simulink model "Engine_TestBench"  (R2017a)
settings: Solver=VariableStepAuto  StartTime=0.0  StopTime=1700  FixedStep=0.01  RelTol=1e-3  EnableMultiTasking=on
PostLoadFcn:
  | , if any(exist('dsrtsu_mdlpostloadfcn', 'file') == [2, 3, 6]), try dsrtsu_mdlpostloadfcn('Execute', bdroot); catch fprintf('Error in PostLoadFcn (dsrtsu_mdlpostloadfcn) for model "%s":\n %s\n', bdroot, lasterr); end, end,
undefined symbols (not defined in the file): air, Engine, env, max_vehicle_rad_air_flow, NeutralGear, ParkGear
libraries: Pneumatic_lib x24, simulink x18, nesl_utility x18, EC2_libraries x2, fl_lib x2
(part 2 of 2)

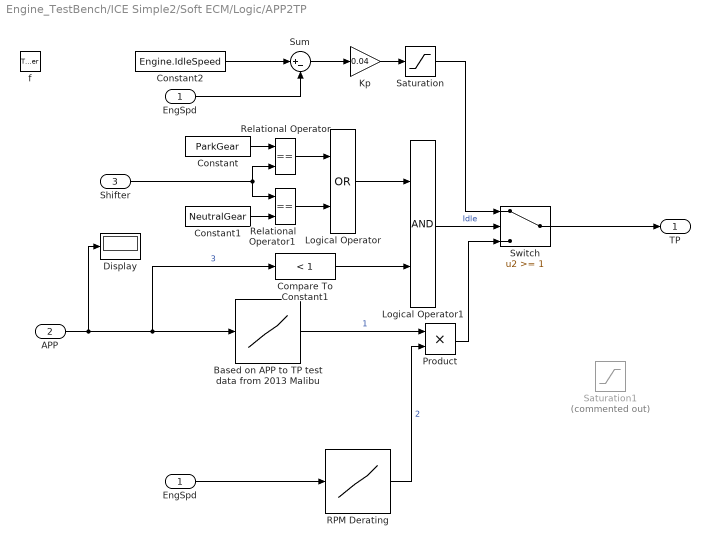
== system Engine_TestBench/ICE Simple2/Soft ECM/Logic/APP2TP ==
  EngSpd : Inport
  APP : Inport  Port=2
  Shifter : Inport  Port=3
  f : TriggerPort  TriggerType=function-call  VariantControl=Variant
      settings: CopyFcn=Stateflow.SLINSF.SimulinkMan.removeBlockPreDeleteFcn  PreDeleteFcn=Stateflow.SLINSF.SimulinkMan.unsafePredeleteFcn
  Based on APP to TP test data from 2013 Malibu : Lookup_n-D  NumberOfTableDimensions=1  BreakpointsForDimension1=[0,1,2,3,4,5,6,7,8,9,10,11,12,13,14,15,16,17,18,19,20,21,22,23,24,25,26,27,28,29,30,31,32,33,34,35,36,37,38,39,40,41,42,43,44,45,46,48,51,55,60,66,100]  Table=[7,12,14,16,16.5,17,18,19,21,23,25,28,29,30,32,35,37,39,41,44,47,48,48.6,49,50,51.5,52,53,53.25,53.5,55,56.75,57,58,60,64,68,72,73,74,75,76,77,77.5,78,80,82,85,87,89.5,91.5,93,100]  InterpMethod=Cubic spline  ExtrapMethod=Cubic spline  UseLastTableValue=on  InputSameDT=on
  Compare To Constant1 : simulink/Logic and Bit Operations/Compare To Constant  relop=<  const=1  OutDataTypeStr=boolean
  Constant : Constant  Value=ParkGear
  Constant1 : Constant  Value=NeutralGear
  Constant2 : Constant  Value=Engine.IdleSpeed
  Display : Display
  "EngSpd " : InportShadow
  Kp : Gain  Gain=0.04
  Logical Operator : Logic  Operator=OR  AllPortsSameDT=off  OutDataTypeStr=boolean
  Logical Operator1 : Logic  AllPortsSameDT=off  OutDataTypeStr=boolean
  Product : Product
  RPM Derating : Lookup_n-D  NumberOfTableDimensions=1  BreakpointsForDimension1=[0 1000 2000 3000 4000 5000 6000 7000]  Table=[1 1 1 1 1 1 1 0]  ExtrapMethod=Clip  UseLastTableValue=on  InternalRulePriority=Speed  RndMeth=Simplest  InputSameDT=on
  Relational Operator : RelationalOperator  Operator===  OutDataTypeStr=boolean  RndMeth=Nearest
  Relational Operator1 : RelationalOperator  Operator===  OutDataTypeStr=boolean  RndMeth=Nearest
  Saturation : Saturate  UpperLimit=100  LowerLimit=0
  Saturation1 : Saturate  Commented=on  UpperLimit=100  LowerLimit=4
  Sum : Sum  Inputs=|+-
  Switch : Switch  Threshold=1
  TP : Outport
  wires:
  Switch/1 -> TP/1
  EngSpd/1 -> RPM Derating/1
  RPM Derating/1 -> Product/2  "2"
  Shifter/1 -> Relational Operator/2, Relational Operator1/1
  Constant/1 -> Relational Operator/1
  Constant1/1 -> Relational Operator1/2
  Relational Operator/1 -> Logical Operator/1
  Relational Operator1/1 -> Logical Operator/2
  Logical Operator/1 -> Logical Operator1/1
  Constant2/1 -> Sum/1
  "EngSpd "/1 -> Sum/2
  Sum/1 -> Kp/1
  Kp/1 -> Saturation/1
  Saturation/1 -> Switch/1
  Logical Operator1/1 -> Switch/2  "Idle"
  Compare To Constant1/1 -> Logical Operator1/2
  APP/1 -> Display/1, Based on APP to TP test data from 2013 Malibu/1, Compare To Constant1/1  "3"
  Product/1 -> Switch/3
  Based on APP to TP test data from 2013 Malibu/1 -> Product/1  "1"

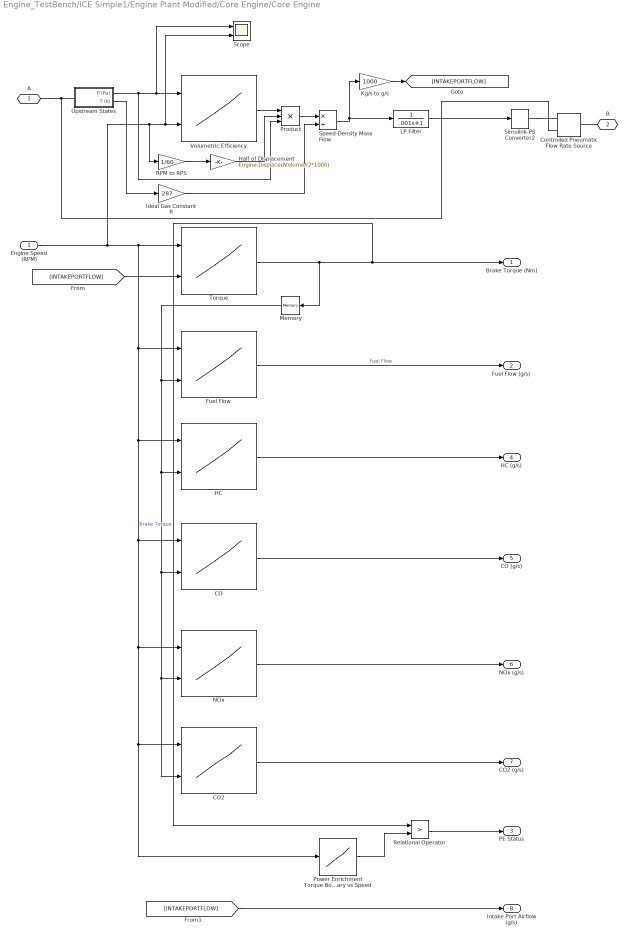
== system Engine_TestBench/ICE Simple1/Engine Plant Modified/Core Engine/Core Engine ==
  Engine Speed (RPM) : Inport
  CO : Lookup2D  RowIndex=Engine.Engine.Emissions.SPEED  ColumnIndex=Engine.Engine.Emissions.TQ  Table=Engine.Engine.Emissions.CO/1000  LookUpMeth=Interpolation-Use End Values
  CO2 : Lookup2D  RowIndex=Engine.Engine.Emissions.SPEED  ColumnIndex=Engine.Engine.Emissions.TQ  Table=Engine.Engine.Emissions.CO2/1000  LookUpMeth=Interpolation-Use End Values
  Controlled Pneumatic Flow Rate Source : Pneumatic_lib/Pneumatic Sources/Controlled Pneumatic Flow Rate Source
  Fuel Flow : Lookup2D  RowIndex=Engine.Engine.FuelFlow.SPEED  ColumnIndex=Engine.Engine.FuelFlow.TQ  Table=Engine.Engine.FuelFlow.FuelFlow  LookUpMeth=Interpolation-Use End Values
  HC : Lookup2D  RowIndex=Engine.Engine.Emissions.SPEED  ColumnIndex=Engine.Engine.Emissions.TQ  Table=Engine.Engine.Emissions.HC/1000  LookUpMeth=Interpolation-Use End Values
  Half of Displacement : Gain  Gain=Engine.DisplacedVolume/(2*1000)
  Ideal Gas Constant R : Gain  Gain=287
  Kg/s to g/s : Gain  Gain=1000
  LP Filter : TransferFcn  Denominator=[.001 1]
  Memory : Memory
  NOx : Lookup2D  RowIndex=Engine.Engine.Emissions.SPEED  ColumnIndex=Engine.Engine.Emissions.TQ  Table=Engine.Engine.Emissions.NOx/1000  LookUpMeth=Interpolation-Use End Values
  Power Enrichment Torque Boundary vs Speed : Lookup_n-D  NumberOfTableDimensions=1  BreakpointsForDimension1=Engine.Engine.PEBound.SPEED  Table=Engine.Engine.PEBound.PEBound  ExtrapMethod=Clip  InternalRulePriority=Speed  RndMeth=Simplest  InputSameDT=on
  Product : Product  Inputs=***
  RPM to RPS : Gain  Gain=1/60
  Relational Operator : RelationalOperator  Operator=>  OutDataTypeStr=boolean  ZeroCross=off  RndMeth=Nearest
  Scope : Scope  NumInputPorts=2
  Simulink-PS Converter2 : nesl_utility/Simulink-PS Converter  PhysicalDomain=network_engine_domain  SubClassName=ps_input  LeftPortType=input  RightPortType=output  PseudoPeriodic=off  Frequencies=[]  NoiseDistribution=none  NoiseParameters=[]  Unit=kg/s  AffineConversion=off  FilteringAndDerivatives=zero  SimscapeFilterOrder=1  InputFilterTimeConstant=.001  UdotUserProvided=0
  Speed-Density Mass Flow : Product  Inputs=*/
  Torque : Lookup2D  RowIndex=Engine.Engine.TQ.SPEED  ColumnIndex=Engine.Engine.TQ.MAF  Table=Engine.Engine.TQ.TQ  LookUpMeth=Interpolation-Use End Values
  Upstream States : Subsystem
  Volumetric Efficiency : Lookup2D  RowIndex=Engine.Engine.VE.MAP  ColumnIndex=Engine.Engine.VE.SPEED  Table=Engine.Engine.VE.VE  LookUpMeth=Interpolation-Use End Values
  A : PMIOPort  Port=1  Side=Left
  B : PMIOPort  Port=2  Side=Right
  Brake Torque (Nm) : Outport
  Fuel Flow (g/s) : Outport  Port=2
  PE Status : Outport  Port=3
  HC (g/s) : Outport  Port=4
  CO (g/s) : Outport  Port=5
  NOx (g/s) : Outport  Port=6
  CO2 (g/s) : Outport  Port=7
  Intake Port Airflow (g/s) : Outport  Port=8
  wires:
  Upstream States/1(P (Pa)) -> Scope/1, Volumetric Efficiency/1, Product/3
  Volumetric Efficiency/1 -> Product/1
  Ideal Gas Constant R/1 -> Speed-Density Mass Flow/2
  Product/1 -> Speed-Density Mass Flow/1
  Upstream States/2(T (K)) -> Ideal Gas Constant R/1
  RPM to RPS/1 -> Half of Displacement/1
  Half of Displacement/1 -> Product/2
  Kg/s to g/s/1 -> [INTAKEPORTFLOW]
  Torque/1 -> Brake Torque (Nm)/1, Relational Operator/1, Memory/1  "Brake Torque"
  [INTAKEPORTFLOW] -> Torque/2
  LP Filter/1 -> Simulink-PS Converter2/1
  Fuel Flow/1 -> Fuel Flow (g/s)/1  "Fuel Flow"
  Engine Speed (RPM)/1 -> Torque/1, Fuel Flow/1, HC/1, CO/1, NOx/1, Power Enrichment Torque Boundary vs Speed/1, CO2/1, Scope/2, Volumetric Efficiency/2, RPM to RPS/1
  Memory/1 -> CO2/2, NOx/2, CO/2, HC/2, Fuel Flow/2
  Power Enrichment Torque Boundary vs Speed/1 -> Relational Operator/2
  Relational Operator/1 -> PE Status/1
  HC/1 -> HC (g/s)/1
  CO/1 -> CO (g/s)/1
  NOx/1 -> NOx (g/s)/1
  CO2/1 -> CO2 (g/s)/1
  [INTAKEPORTFLOW] -> Intake Port Airflow (g/s)/1
  Speed-Density Mass Flow/1 -> LP Filter/1, Kg/s to g/s/1
  connections:
  Upstream States/LConn1 -- A/RConn1 -- Controlled Pneumatic Flow Rate Source/RConn1
  B/RConn1 -- Controlled Pneumatic Flow Rate Source/LConn1
  Simulink-PS Converter2/RConn1 -- Controlled Pneumatic Flow Rate Source/RConn2

== system Engine_TestBench/ICE Simple1/Engine Plant Modified/Core Engine/Crank Process/function ==
  EngSpd : Inport
  f : TriggerPort  TriggerType=function-call  VariantControl=Variant
      settings: CopyFcn=Stateflow.SLINSF.SimulinkMan.removeBlockPreDeleteFcn  PreDeleteFcn=Stateflow.SLINSF.SimulinkMan.unsafePredeleteFcn
  1-D Lookup Table : Lookup_n-D  NumberOfTableDimensions=1  BreakpointsForDimension1=[0 50 120 210 300 320 340 350 400]  Table="[90 90 90 10 5 5  5 5 5]"  InternalRulePriority=Speed  RndMeth=Simplest  InputSameDT=on
  Sine Wave : Sin  Amplitude=20  Frequency=41.88
  Sum : Sum
  CrankTrq : Outport
  wires:
  1-D Lookup Table/1 -> Sum/1
  EngSpd/1 -> 1-D Lookup Table/1
  Sum/1 -> CrankTrq/1
  Sine Wave/1 -> Sum/2

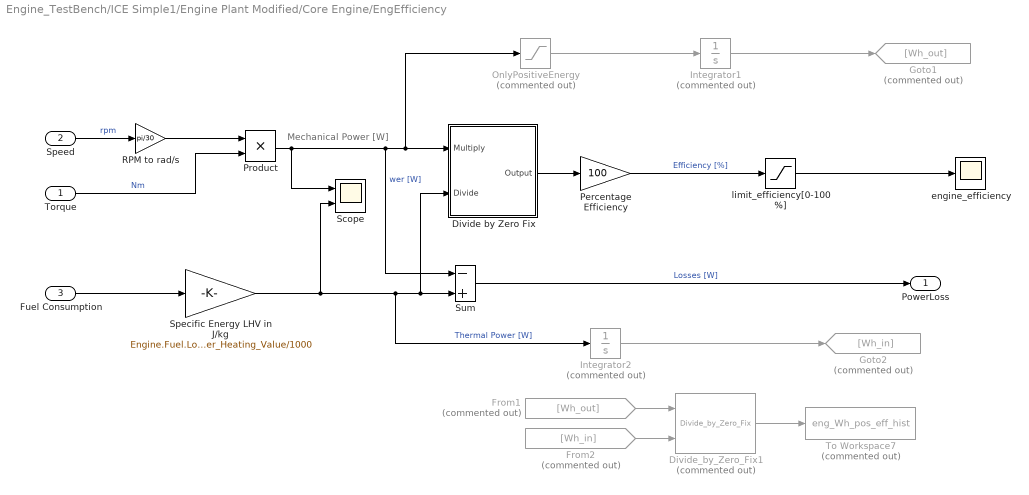
== system Engine_TestBench/ICE Simple1/Engine Plant Modified/Core Engine/EngEfficiency ==
  note: Mechanical Power [W]
  Torque : Inport
  Speed : Inport  Port=2
  Fuel Consumption : Inport  Port=3
  Divide by Zero Fix : Subsystem
  Divide_by_Zero_Fix1 : EC2_libraries/Divide_by_Zero_Fix  Commented=on
  From1 : From  Commented=on  GotoTag=Wh_out
  From2 : From  Commented=on  GotoTag=Wh_in
  Goto1 : Goto  Commented=on  GotoTag=Wh_out
  Goto2 : Goto  Commented=on  GotoTag=Wh_in
  Integrator1 : Integrator  Commented=on  LimitOutput=on  LowerSaturationLimit=0
  Integrator2 : Integrator  Commented=on  LimitOutput=on  LowerSaturationLimit=0
  OnlyPositiveEnergy : Saturate  Commented=on  UpperLimit=inf  LowerLimit=0
  Percentage Efficiency : Gain  Gain=100
  Product : Product  RndMeth=Zero
  "RPM to rad/s " : Gain  Gain=pi/30
  Scope : Scope  NumInputPorts=2
  Specific Energy LHV in J/kg : Gain  Gain=Engine.Fuel.Lower_Heating_Value/1000
  Sum : Sum  Inputs=-+
  To Workspace7 : ToWorkspace  Commented=on  VariableName=eng_Wh_pos_eff_hist  SampleTime=-1
      settings: Decimation=WORKSPACE_DECIMATION
  engine_efficiency : Scope
  limit_efficiency[0-100%] : Saturate  UpperLimit=100  LowerLimit=0
  PowerLoss : Outport
  wires:
  limit_efficiency[0-100%]/1 -> engine_efficiency/1
  Sum/1 -> PowerLoss/1  "Losses [W]"
  Fuel Consumption/1 -> Specific Energy LHV in J/kg/1
  Specific Energy LHV in J/kg/1 -> Divide by Zero Fix/2(Divide), Sum/2, Integrator2/1, Scope/2  "Thermal Power [W]"
  Torque/1 -> Product/2  "Nm"
  Speed/1 -> "RPM to rad/s "/1  "rpm"
  Percentage Efficiency/1 -> limit_efficiency[0-100%]/1  "Efficiency [%]"
  Divide by Zero Fix/1(Output) -> Percentage Efficiency/1
  Product/1 -> Scope/1, Divide by Zero Fix/1(Multiply), OnlyPositiveEnergy/1, Sum/1  "wer [W]"
  Divide_by_Zero_Fix1/1 -> To Workspace7/1
  From1/1 -> Divide_by_Zero_Fix1/1
  From2/1 -> Divide_by_Zero_Fix1/2
  Integrator1/1 -> Goto1/1
  OnlyPositiveEnergy/1 -> Integrator1/1
  Integrator2/1 -> Goto2/1
  "RPM to rad/s "/1 -> Product/1

== system Engine_TestBench/ICE Simple1/Engine Plant Modified/Core Engine/EngineThermal ==
  note: Temp Delta C deg
  PowerLoss : Inport
  Divide : Product  Inputs=*/
  Divide1 : Product  Inputs=**
  Engine Mass : Constant  Value=Engine.Mass
  Memory : Memory  X0=Engine.Init_T_amb
  Memory1 : Memory
  Product : Product  RndMeth=Zero
  Specific Heat Cap Aluminum : Constant  Value=Engine.Specific_Heat
  Sum : Sum  Inputs=|++
  Sum1 : Sum  Inputs=|+-
  tloop : Constant  Value=0.01
  Temp[degC] : Outport
  tag scope: Heat_Transfer_Eng=global
  wires:
  Memory1/1 -> Sum1/2
  Divide1/1 -> Divide/1  "J"
  Sum1/1 -> Divide1/2
  Memory/1 -> Sum/2
  PowerLoss/1 -> Sum1/1, [Heat_Transfer_Eng]  "J/s"
  Engine Mass/1 -> Product/1  "kg"
  Specific Heat Cap Aluminum/1 -> Product/2  "J/kg*K"
  Product/1 -> Divide/2
  Sum/1 -> Memory/1, Temp[degC]/1
  Divide/1 -> Sum/1
  tloop/1 -> Divide1/1
  [Heat_Reject_Eng] -> Memory1/1

== system Engine_TestBench/ICE Simple1/Engine Plant Modified/Core Engine/Intake Manifold ==
  note: 3.4
  note: 2.4
  Heat-Transfer Neglected : fl_lib/Thermal/Thermal Elements/Perfect Insulator  T_specify=off  T_priority=None  T=0 K  T_nominal_specify=off  T_nominal_unit=K  T_nominal_value=1
      settings: SourceProductName=Simscape
  Intake Manifold Volume : Pneumatic_lib/Pneumatic Elements/Constant Volume Pneumatic Chamber  Volume=3.6 l  pressure_specify=on  pressure_priority=High  pressure=26 kPa  pressure_nominal_specify=off  pressure_nominal_unit=Pa  pressure_nominal_value=1  temperature_specify=on  temperature_priority=High  temperature=20 K  temperature_nominal_specify=off  temperature_nominal_unit=K  temperature_nominal_value=1  gas_flow_specify=off  gas_flow_priority=High  gas_flow=0 kg/s  gas_flow_nominal_specify=off  gas_flow_nominal_unit=kg/s  gas_flow_nominal_value=1  heat_flow_specify=off  heat_flow_priority=High  heat_flow=0 J/s  heat_flow_nominal_specify=off  heat_flow_nominal_unit=J/s  heat_flow_nominal_value=1  heat_exch_flow_specify=off  heat_exch_flow_priority=High  heat_exch_flow=0 J/s  heat_exch_flow_nominal_specify=off  heat_exch_flow_nominal_unit=J/s  heat_exch_flow_nominal_value=1
  Intake Manifold Volume1 : Pneumatic_lib/Pneumatic Elements/Constant Volume Pneumatic Chamber  Commented=on  Volume=Engine.IntakeManifold.Volume l  pressure_specify=on  pressure_priority=High  pressure=26 kPa  pressure_nominal_specify=off  pressure_nominal_unit=Pa  pressure_nominal_value=1  temperature_specify=on  temperature_priority=High  temperature=20 K  temperature_nominal_specify=off  temperature_nominal_unit=K  temperature_nominal_value=1  gas_flow_specify=off  gas_flow_priority=High  gas_flow=0 kg/s  gas_flow_nominal_specify=off  gas_flow_nominal_unit=kg/s  gas_flow_nominal_value=1  heat_flow_specify=off  heat_flow_priority=High  heat_flow=0 J/s  heat_flow_nominal_specify=off  heat_flow_nominal_unit=J/s  heat_flow_nominal_value=1  heat_exch_flow_specify=off  heat_exch_flow_priority=High  heat_exch_flow=0 J/s  heat_exch_flow_nominal_specify=off  heat_exch_flow_nominal_unit=J/s  heat_exch_flow_nominal_value=1
  Node Potential Sensor : Subsystem
  A : PMIOPort  Port=1  Side=Left
  MAP : Outport
  MAT : Outport  Port=2
  wires:
  Node Potential Sensor/1(P (KPa)) -> MAP/1
  Node Potential Sensor/2(T (C)) -> MAT/1
  connections:
  Node Potential Sensor/LConn1 -- A/RConn1 -- Intake Manifold Volume/LConn1
  Heat-Transfer Neglected/LConn1 -- Intake Manifold Volume/LConn2

== system Engine_TestBench/ICE Simple1/Engine Plant Modified/Core Engine/Throttle Body ==
  Throttle Position % CMD : Inport
  CA vs TP : Lookup  InputValues=Engine.Throttle.CA.TPP  Table=Engine.Throttle.CA.CA  LookUpMeth=Interpolation-Use End Values
  ETC Actuator Dynamics : TransferFcn  Denominator=[0.1 1]
  PS-Simulink Converter : nesl_utility/PS-Simulink Converter  PhysicalDomain=network_engine_domain  SubClassName=ps_output  LeftPortType=input  RightPortType=output  PseudoPeriodic=off  Frequencies=[]  Unit=g/s  AffineConversion=off
  PS-Simulink Converter1 : nesl_utility/PS-Simulink Converter  PhysicalDomain=network_engine_domain  SubClassName=ps_output  LeftPortType=input  RightPortType=output  PseudoPeriodic=off  Frequencies=[]  Unit=J/s  AffineConversion=off
  Pneumatic Mass & Heat Flow Sensor : Pneumatic_lib/Pneumatic Sensors/Pneumatic Mass & Heat Flow Sensor
  Simulink-PS Converter : nesl_utility/Simulink-PS Converter  PhysicalDomain=network_engine_domain  SubClassName=ps_input  LeftPortType=input  RightPortType=output  PseudoPeriodic=off  Frequencies=[]  NoiseDistribution=none  NoiseParameters=[]  Unit=m^2  AffineConversion=off  FilteringAndDerivatives=zero  SimscapeFilterOrder=1  InputFilterTimeConstant=.001  UdotUserProvided=0
  Terminator : Terminator
  Throttle Throat : Pneumatic_lib/Pneumatic Elements/Variable Area Pneumatic Orifice  Cd=0.82  Area0=1e-12 m^2  G_specify=off  G_priority=High  G=0 kg/s  G_nominal_specify=off  G_nominal_unit=kg/s  G_nominal_value=1  Q1_specify=off  Q1_priority=High  Q1=0 J/s  Q1_nominal_specify=off  Q1_nominal_unit=J/s  Q1_nominal_value=1  Q2_specify=off  Q2_priority=High  Q2=0 J/s  Q2_nominal_specify=off  Q2_nominal_unit=J/s  Q2_nominal_value=1  p1_specify=off  p1_priority=High  p1=1e+5 Pa  p1_nominal_specify=off  p1_nominal_unit=Pa  p1_nominal_value=1  p2_specify=off  p2_priority=High  p2=1e+5 Pa  p2_nominal_specify=off  p2_nominal_unit=Pa  p2_nominal_value=1  T1_specify=off  T1_priority=High  T1=300 K  T1_nominal_specify=off  T1_nominal_unit=K  T1_nominal_value=1  T2_specify=off  T2_priority=High  T2=300 K  T2_nominal_specify=off  T2_nominal_unit=K  T2_nominal_value=1
  B : PMIOPort  Port=1  Side=Right
  A : PMIOPort  Port=2  Side=Left
  Throttle Flow kg/s : Outport
  Throttle Position % : Outport  Port=2
  wires:
  ETC Actuator Dynamics/1 -> CA vs TP/1, Throttle Position %/1
  CA vs TP/1 -> Simulink-PS Converter/1
  PS-Simulink Converter/1 -> Throttle Flow kg/s/1
  PS-Simulink Converter1/1 -> Terminator/1
  Throttle Position % CMD/1 -> ETC Actuator Dynamics/1
  connections:
  Simulink-PS Converter/RConn1 -- Throttle Throat/LConn2
  Throttle Throat/LConn1 -- A/RConn1
  Pneumatic Mass & Heat Flow Sensor/RConn2 -- PS-Simulink Converter/LConn1
  Pneumatic Mass & Heat Flow Sensor/RConn3 -- PS-Simulink Converter1/LConn1
  Throttle Throat/RConn1 -- Pneumatic Mass & Heat Flow Sensor/LConn1
  Pneumatic Mass & Heat Flow Sensor/RConn1 -- B/RConn1

== system Engine_TestBench/ICE Simple1/Engine Plant Modified/Radiator/Divide by Zero Fix ==
  Multiply : Inport
  Divide : Inport  Port=2
  Compare To Zero : simulink/Logic and Bit Operations/Compare To Zero  relop===  OutDataTypeStr=boolean
  Constant1 : Constant  Value=0
  Constant2 : Constant
  Product2 : Product  Inputs=/*  SaturateOnIntegerOverflow=on  InputSameDT=on  OutDataTypeStr=Inherit: Same as first input
  Switch : Switch  Threshold=1
  Switch1 : Switch  Threshold=1
  Output : Outport
  wires:
  Multiply/1 -> Product2/2
  Switch1/1 -> Output/1
  Constant1/1 -> Switch1/1
  Product2/1 -> Switch1/3
  Switch/1 -> Product2/1
  Divide/1 -> Switch/3, Compare To Zero/1
  Constant2/1 -> Switch/1
  Compare To Zero/1 -> Switch1/2, Switch/2

== system Engine_TestBench/ICE Simple1/Soft ECM/Fuel Consumption/Divide by Zero Fix ==
  Divide : Inport
  Multiply : Inport  Port=2
  Compare To Zero : simulink/Logic and Bit Operations/Compare To Zero  relop===  OutDataTypeStr=boolean
  Constant1 : Constant  Value=0
  Constant2 : Constant
  Product2 : Product  Inputs=/*  SaturateOnIntegerOverflow=on  InputSameDT=on  OutDataTypeStr=Inherit: Same as first input
  Switch : Switch  Threshold=1
  Switch1 : Switch  Threshold=1
  Output : Outport
  wires:
  Multiply/1 -> Product2/2
  Switch1/1 -> Output/1
  Constant1/1 -> Switch1/1
  Product2/1 -> Switch1/3
  Switch/1 -> Product2/1
  Divide/1 -> Compare To Zero/1, Switch/3
  Constant2/1 -> Switch/1
  Compare To Zero/1 -> Switch1/2, Switch/2

== system Engine_TestBench/ICE Simple1/Soft ECM/Fuel Consumption/Divide by Zero Fix1 ==
  Divide : Inport
  Multiply : Inport  Port=2
  Compare To Zero : simulink/Logic and Bit Operations/Compare To Zero  relop===  OutDataTypeStr=boolean
  Constant1 : Constant  Value=0
  Constant2 : Constant
  Product2 : Product  Inputs=/*  SaturateOnIntegerOverflow=on  InputSameDT=on  OutDataTypeStr=Inherit: Same as first input
  Switch : Switch  Threshold=1
  Switch1 : Switch  Threshold=1
  Output : Outport
  wires:
  Compare To Zero/1 -> Switch/2, Switch1/2
  Constant2/1 -> Switch/1
  Divide/1 -> Compare To Zero/1, Switch/3
  Switch/1 -> Product2/1
  Product2/1 -> Switch1/3
  Constant1/1 -> Switch1/1
  Switch1/1 -> Output/1
  Multiply/1 -> Product2/2

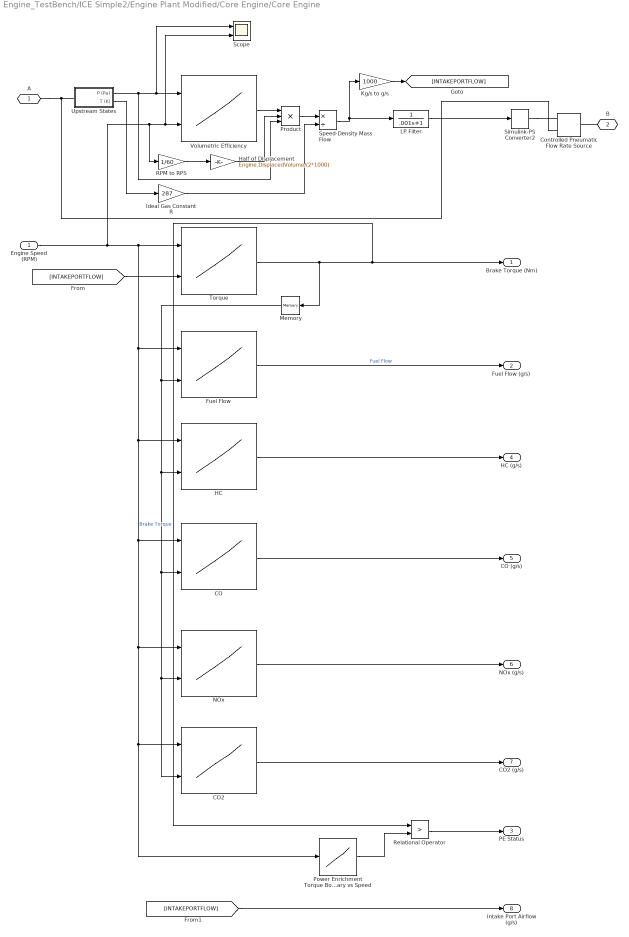
== system Engine_TestBench/ICE Simple2/Engine Plant Modified/Core Engine/Core Engine ==
  Engine Speed (RPM) : Inport
  CO : Lookup2D  RowIndex=Engine.Engine.Emissions.SPEED  ColumnIndex=Engine.Engine.Emissions.TQ  Table=Engine.Engine.Emissions.CO/1000  LookUpMeth=Interpolation-Use End Values
  CO2 : Lookup2D  RowIndex=Engine.Engine.Emissions.SPEED  ColumnIndex=Engine.Engine.Emissions.TQ  Table=Engine.Engine.Emissions.CO2/1000  LookUpMeth=Interpolation-Use End Values
  Controlled Pneumatic Flow Rate Source : Pneumatic_lib/Pneumatic Sources/Controlled Pneumatic Flow Rate Source
  Fuel Flow : Lookup2D  RowIndex=Engine.Engine.FuelFlow.SPEED  ColumnIndex=Engine.Engine.FuelFlow.TQ  Table=Engine.Engine.FuelFlow.FuelFlow  LookUpMeth=Interpolation-Use End Values
  HC : Lookup2D  RowIndex=Engine.Engine.Emissions.SPEED  ColumnIndex=Engine.Engine.Emissions.TQ  Table=Engine.Engine.Emissions.HC/1000  LookUpMeth=Interpolation-Use End Values
  Half of Displacement : Gain  Gain=Engine.DisplacedVolume/(2*1000)
  Ideal Gas Constant R : Gain  Gain=287
  Kg/s to g/s : Gain  Gain=1000
  LP Filter : TransferFcn  Denominator=[.001 1]
  Memory : Memory
  NOx : Lookup2D  RowIndex=Engine.Engine.Emissions.SPEED  ColumnIndex=Engine.Engine.Emissions.TQ  Table=Engine.Engine.Emissions.NOx/1000  LookUpMeth=Interpolation-Use End Values
  Power Enrichment Torque Boundary vs Speed : Lookup_n-D  NumberOfTableDimensions=1  BreakpointsForDimension1=Engine.Engine.PEBound.SPEED  Table=Engine.Engine.PEBound.PEBound  ExtrapMethod=Clip  InternalRulePriority=Speed  RndMeth=Simplest  InputSameDT=on
  Product : Product  Inputs=***
  RPM to RPS : Gain  Gain=1/60
  Relational Operator : RelationalOperator  Operator=>  OutDataTypeStr=boolean  ZeroCross=off  RndMeth=Nearest
  Scope : Scope  NumInputPorts=2
  Simulink-PS Converter2 : nesl_utility/Simulink-PS Converter  PhysicalDomain=network_engine_domain  SubClassName=ps_input  LeftPortType=input  RightPortType=output  PseudoPeriodic=off  Frequencies=[]  NoiseDistribution=none  NoiseParameters=[]  Unit=kg/s  AffineConversion=off  FilteringAndDerivatives=zero  SimscapeFilterOrder=1  InputFilterTimeConstant=.001  UdotUserProvided=0
  Speed-Density Mass Flow : Product  Inputs=*/
  Torque : Lookup2D  RowIndex=Engine.Engine.TQ.SPEED  ColumnIndex=Engine.Engine.TQ.MAF  Table=Engine.Engine.TQ.TQ  LookUpMeth=Interpolation-Use End Values
  Upstream States : Subsystem
  Volumetric Efficiency : Lookup2D  RowIndex=Engine.Engine.VE.MAP  ColumnIndex=Engine.Engine.VE.SPEED  Table=Engine.Engine.VE.VE  LookUpMeth=Interpolation-Use End Values
  A : PMIOPort  Port=1  Side=Left
  B : PMIOPort  Port=2  Side=Right
  Brake Torque (Nm) : Outport
  Fuel Flow (g/s) : Outport  Port=2
  PE Status : Outport  Port=3
  HC (g/s) : Outport  Port=4
  CO (g/s) : Outport  Port=5
  NOx (g/s) : Outport  Port=6
  CO2 (g/s) : Outport  Port=7
  Intake Port Airflow (g/s) : Outport  Port=8
  wires:
  Upstream States/1(P (Pa)) -> Scope/1, Volumetric Efficiency/1, Product/3
  Volumetric Efficiency/1 -> Product/1
  Ideal Gas Constant R/1 -> Speed-Density Mass Flow/2
  Product/1 -> Speed-Density Mass Flow/1
  Upstream States/2(T (K)) -> Ideal Gas Constant R/1
  RPM to RPS/1 -> Half of Displacement/1
  Half of Displacement/1 -> Product/2
  Kg/s to g/s/1 -> [INTAKEPORTFLOW]
  Torque/1 -> Brake Torque (Nm)/1, Relational Operator/1, Memory/1  "Brake Torque"
  [INTAKEPORTFLOW] -> Torque/2
  LP Filter/1 -> Simulink-PS Converter2/1
  Fuel Flow/1 -> Fuel Flow (g/s)/1  "Fuel Flow"
  Engine Speed (RPM)/1 -> Torque/1, Fuel Flow/1, HC/1, CO/1, NOx/1, Power Enrichment Torque Boundary vs Speed/1, CO2/1, Scope/2, Volumetric Efficiency/2, RPM to RPS/1
  Memory/1 -> CO2/2, NOx/2, CO/2, HC/2, Fuel Flow/2
  Power Enrichment Torque Boundary vs Speed/1 -> Relational Operator/2
  Relational Operator/1 -> PE Status/1
  HC/1 -> HC (g/s)/1
  CO/1 -> CO (g/s)/1
  NOx/1 -> NOx (g/s)/1
  CO2/1 -> CO2 (g/s)/1
  [INTAKEPORTFLOW] -> Intake Port Airflow (g/s)/1
  Speed-Density Mass Flow/1 -> LP Filter/1, Kg/s to g/s/1
  connections:
  Upstream States/LConn1 -- A/RConn1 -- Controlled Pneumatic Flow Rate Source/RConn1
  B/RConn1 -- Controlled Pneumatic Flow Rate Source/LConn1
  Simulink-PS Converter2/RConn1 -- Controlled Pneumatic Flow Rate Source/RConn2

== system Engine_TestBench/ICE Simple2/Engine Plant Modified/Core Engine/Crank Process/function ==
  EngSpd : Inport
  f : TriggerPort  TriggerType=function-call  VariantControl=Variant
      settings: CopyFcn=Stateflow.SLINSF.SimulinkMan.removeBlockPreDeleteFcn  PreDeleteFcn=Stateflow.SLINSF.SimulinkMan.unsafePredeleteFcn
  1-D Lookup Table : Lookup_n-D  NumberOfTableDimensions=1  BreakpointsForDimension1=[0 50 120 210 300 320 340 350 400]  Table="[90 90 90 10 5 5  5 5 5]"  InternalRulePriority=Speed  RndMeth=Simplest  InputSameDT=on
  Sine Wave : Sin  Amplitude=20  Frequency=41.88
  Sum : Sum
  CrankTrq : Outport
  wires:
  1-D Lookup Table/1 -> Sum/1
  EngSpd/1 -> 1-D Lookup Table/1
  Sum/1 -> CrankTrq/1
  Sine Wave/1 -> Sum/2

== system Engine_TestBench/ICE Simple2/Engine Plant Modified/Core Engine/EngEfficiency ==
  note: Mechanical Power [W]
  Torque : Inport
  Speed : Inport  Port=2
  Fuel Consumption : Inport  Port=3
  Divide by Zero Fix : Subsystem
  Divide_by_Zero_Fix1 : EC2_libraries/Divide_by_Zero_Fix  Commented=on
  From1 : From  Commented=on  GotoTag=Wh_out
  From2 : From  Commented=on  GotoTag=Wh_in
  Goto1 : Goto  Commented=on  GotoTag=Wh_out
  Goto2 : Goto  Commented=on  GotoTag=Wh_in
  Integrator1 : Integrator  Commented=on  LimitOutput=on  LowerSaturationLimit=0
  Integrator2 : Integrator  Commented=on  LimitOutput=on  LowerSaturationLimit=0
  OnlyPositiveEnergy : Saturate  Commented=on  UpperLimit=inf  LowerLimit=0
  Percentage Efficiency : Gain  Gain=100
  Product : Product  RndMeth=Zero
  "RPM to rad/s " : Gain  Gain=pi/30
  Scope : Scope  NumInputPorts=2
  Specific Energy LHV in J/kg : Gain  Gain=Engine.Fuel.Lower_Heating_Value/1000
  Sum : Sum  Inputs=-+
  To Workspace7 : ToWorkspace  Commented=on  VariableName=eng_Wh_pos_eff_hist  SampleTime=-1
      settings: Decimation=WORKSPACE_DECIMATION
  engine_efficiency : Scope
  limit_efficiency[0-100%] : Saturate  UpperLimit=100  LowerLimit=0
  PowerLoss : Outport
  wires:
  limit_efficiency[0-100%]/1 -> engine_efficiency/1
  Sum/1 -> PowerLoss/1  "Losses [W]"
  Fuel Consumption/1 -> Specific Energy LHV in J/kg/1
  Specific Energy LHV in J/kg/1 -> Divide by Zero Fix/2(Divide), Sum/2, Integrator2/1, Scope/2  "Thermal Power [W]"
  Torque/1 -> Product/2  "Nm"
  Speed/1 -> "RPM to rad/s "/1  "rpm"
  Percentage Efficiency/1 -> limit_efficiency[0-100%]/1  "Efficiency [%]"
  Divide by Zero Fix/1(Output) -> Percentage Efficiency/1
  Product/1 -> Scope/1, Divide by Zero Fix/1(Multiply), OnlyPositiveEnergy/1, Sum/1  "wer [W]"
  Divide_by_Zero_Fix1/1 -> To Workspace7/1
  From1/1 -> Divide_by_Zero_Fix1/1
  From2/1 -> Divide_by_Zero_Fix1/2
  Integrator1/1 -> Goto1/1
  OnlyPositiveEnergy/1 -> Integrator1/1
  Integrator2/1 -> Goto2/1
  "RPM to rad/s "/1 -> Product/1

== system Engine_TestBench/ICE Simple2/Engine Plant Modified/Core Engine/EngineThermal ==
  note: Temp Delta C deg
  PowerLoss : Inport
  Divide : Product  Inputs=*/
  Divide1 : Product  Inputs=**
  Engine Mass : Constant  Value=Engine.Mass
  Memory : Memory  X0=Engine.Init_T_amb
  Memory1 : Memory
  Product : Product  RndMeth=Zero
  Specific Heat Cap Aluminum : Constant  Value=Engine.Specific_Heat
  Sum : Sum  Inputs=|++
  Sum1 : Sum  Inputs=|+-
  tloop : Constant  Value=0.01
  Temp[degC] : Outport
  tag scope: Heat_Transfer_Eng=global
  wires:
  Memory1/1 -> Sum1/2
  Divide1/1 -> Divide/1  "J"
  Sum1/1 -> Divide1/2
  Memory/1 -> Sum/2
  PowerLoss/1 -> Sum1/1, [Heat_Transfer_Eng]  "J/s"
  Engine Mass/1 -> Product/1  "kg"
  Specific Heat Cap Aluminum/1 -> Product/2  "J/kg*K"
  Product/1 -> Divide/2
  Sum/1 -> Memory/1, Temp[degC]/1
  Divide/1 -> Sum/1
  tloop/1 -> Divide1/1
  [Heat_Reject_Eng] -> Memory1/1

== system Engine_TestBench/ICE Simple2/Engine Plant Modified/Core Engine/Intake Manifold ==
  note: 3.4
  note: 2.4
  Heat-Transfer Neglected : fl_lib/Thermal/Thermal Elements/Perfect Insulator  T_specify=off  T_priority=None  T=0 K  T_nominal_specify=off  T_nominal_unit=K  T_nominal_value=1
      settings: SourceProductName=Simscape
  Intake Manifold Volume : Pneumatic_lib/Pneumatic Elements/Constant Volume Pneumatic Chamber  Volume=3.6 l  pressure_specify=on  pressure_priority=High  pressure=26 kPa  pressure_nominal_specify=off  pressure_nominal_unit=Pa  pressure_nominal_value=1  temperature_specify=on  temperature_priority=High  temperature=20 K  temperature_nominal_specify=off  temperature_nominal_unit=K  temperature_nominal_value=1  gas_flow_specify=off  gas_flow_priority=High  gas_flow=0 kg/s  gas_flow_nominal_specify=off  gas_flow_nominal_unit=kg/s  gas_flow_nominal_value=1  heat_flow_specify=off  heat_flow_priority=High  heat_flow=0 J/s  heat_flow_nominal_specify=off  heat_flow_nominal_unit=J/s  heat_flow_nominal_value=1  heat_exch_flow_specify=off  heat_exch_flow_priority=High  heat_exch_flow=0 J/s  heat_exch_flow_nominal_specify=off  heat_exch_flow_nominal_unit=J/s  heat_exch_flow_nominal_value=1
  Intake Manifold Volume1 : Pneumatic_lib/Pneumatic Elements/Constant Volume Pneumatic Chamber  Commented=on  Volume=Engine.IntakeManifold.Volume l  pressure_specify=on  pressure_priority=High  pressure=26 kPa  pressure_nominal_specify=off  pressure_nominal_unit=Pa  pressure_nominal_value=1  temperature_specify=on  temperature_priority=High  temperature=20 K  temperature_nominal_specify=off  temperature_nominal_unit=K  temperature_nominal_value=1  gas_flow_specify=off  gas_flow_priority=High  gas_flow=0 kg/s  gas_flow_nominal_specify=off  gas_flow_nominal_unit=kg/s  gas_flow_nominal_value=1  heat_flow_specify=off  heat_flow_priority=High  heat_flow=0 J/s  heat_flow_nominal_specify=off  heat_flow_nominal_unit=J/s  heat_flow_nominal_value=1  heat_exch_flow_specify=off  heat_exch_flow_priority=High  heat_exch_flow=0 J/s  heat_exch_flow_nominal_specify=off  heat_exch_flow_nominal_unit=J/s  heat_exch_flow_nominal_value=1
  Node Potential Sensor : Subsystem
  A : PMIOPort  Port=1  Side=Left
  MAP : Outport
  MAT : Outport  Port=2
  wires:
  Node Potential Sensor/1(P (KPa)) -> MAP/1
  Node Potential Sensor/2(T (C)) -> MAT/1
  connections:
  Node Potential Sensor/LConn1 -- A/RConn1 -- Intake Manifold Volume/LConn1
  Heat-Transfer Neglected/LConn1 -- Intake Manifold Volume/LConn2

== system Engine_TestBench/ICE Simple2/Engine Plant Modified/Core Engine/Throttle Body ==
  Throttle Position % CMD : Inport
  CA vs TP : Lookup  InputValues=Engine.Throttle.CA.TPP  Table=Engine.Throttle.CA.CA  LookUpMeth=Interpolation-Use End Values
  ETC Actuator Dynamics : TransferFcn  Denominator=[0.1 1]
  PS-Simulink Converter : nesl_utility/PS-Simulink Converter  PhysicalDomain=network_engine_domain  SubClassName=ps_output  LeftPortType=input  RightPortType=output  PseudoPeriodic=off  Frequencies=[]  Unit=g/s  AffineConversion=off
  PS-Simulink Converter1 : nesl_utility/PS-Simulink Converter  PhysicalDomain=network_engine_domain  SubClassName=ps_output  LeftPortType=input  RightPortType=output  PseudoPeriodic=off  Frequencies=[]  Unit=J/s  AffineConversion=off
  Pneumatic Mass & Heat Flow Sensor : Pneumatic_lib/Pneumatic Sensors/Pneumatic Mass & Heat Flow Sensor
  Simulink-PS Converter : nesl_utility/Simulink-PS Converter  PhysicalDomain=network_engine_domain  SubClassName=ps_input  LeftPortType=input  RightPortType=output  PseudoPeriodic=off  Frequencies=[]  NoiseDistribution=none  NoiseParameters=[]  Unit=m^2  AffineConversion=off  FilteringAndDerivatives=zero  SimscapeFilterOrder=1  InputFilterTimeConstant=.001  UdotUserProvided=0
  Terminator : Terminator
  Throttle Throat : Pneumatic_lib/Pneumatic Elements/Variable Area Pneumatic Orifice  Cd=0.82  Area0=1e-12 m^2  G_specify=off  G_priority=High  G=0 kg/s  G_nominal_specify=off  G_nominal_unit=kg/s  G_nominal_value=1  Q1_specify=off  Q1_priority=High  Q1=0 J/s  Q1_nominal_specify=off  Q1_nominal_unit=J/s  Q1_nominal_value=1  Q2_specify=off  Q2_priority=High  Q2=0 J/s  Q2_nominal_specify=off  Q2_nominal_unit=J/s  Q2_nominal_value=1  p1_specify=off  p1_priority=High  p1=1e+5 Pa  p1_nominal_specify=off  p1_nominal_unit=Pa  p1_nominal_value=1  p2_specify=off  p2_priority=High  p2=1e+5 Pa  p2_nominal_specify=off  p2_nominal_unit=Pa  p2_nominal_value=1  T1_specify=off  T1_priority=High  T1=300 K  T1_nominal_specify=off  T1_nominal_unit=K  T1_nominal_value=1  T2_specify=off  T2_priority=High  T2=300 K  T2_nominal_specify=off  T2_nominal_unit=K  T2_nominal_value=1
  B : PMIOPort  Port=1  Side=Right
  A : PMIOPort  Port=2  Side=Left
  Throttle Flow kg/s : Outport
  Throttle Position % : Outport  Port=2
  wires:
  ETC Actuator Dynamics/1 -> CA vs TP/1, Throttle Position %/1
  CA vs TP/1 -> Simulink-PS Converter/1
  PS-Simulink Converter/1 -> Throttle Flow kg/s/1
  PS-Simulink Converter1/1 -> Terminator/1
  Throttle Position % CMD/1 -> ETC Actuator Dynamics/1
  connections:
  Simulink-PS Converter/RConn1 -- Throttle Throat/LConn2
  Throttle Throat/LConn1 -- A/RConn1
  Pneumatic Mass & Heat Flow Sensor/RConn2 -- PS-Simulink Converter/LConn1
  Pneumatic Mass & Heat Flow Sensor/RConn3 -- PS-Simulink Converter1/LConn1
  Throttle Throat/RConn1 -- Pneumatic Mass & Heat Flow Sensor/LConn1
  Pneumatic Mass & Heat Flow Sensor/RConn1 -- B/RConn1

== system Engine_TestBench/ICE Simple2/Engine Plant Modified/Radiator/Divide by Zero Fix ==
  Multiply : Inport
  Divide : Inport  Port=2
  Compare To Zero : simulink/Logic and Bit Operations/Compare To Zero  relop===  OutDataTypeStr=boolean
  Constant1 : Constant  Value=0
  Constant2 : Constant
  Product2 : Product  Inputs=/*  SaturateOnIntegerOverflow=on  InputSameDT=on  OutDataTypeStr=Inherit: Same as first input
  Switch : Switch  Threshold=1
  Switch1 : Switch  Threshold=1
  Output : Outport
  wires:
  Multiply/1 -> Product2/2
  Switch1/1 -> Output/1
  Constant1/1 -> Switch1/1
  Product2/1 -> Switch1/3
  Switch/1 -> Product2/1
  Divide/1 -> Switch/3, Compare To Zero/1
  Constant2/1 -> Switch/1
  Compare To Zero/1 -> Switch1/2, Switch/2

== system Engine_TestBench/ICE Simple2/Soft ECM/Fuel Consumption/Divide by Zero Fix ==
  Divide : Inport
  Multiply : Inport  Port=2
  Compare To Zero : simulink/Logic and Bit Operations/Compare To Zero  relop===  OutDataTypeStr=boolean
  Constant1 : Constant  Value=0
  Constant2 : Constant
  Product2 : Product  Inputs=/*  SaturateOnIntegerOverflow=on  InputSameDT=on  OutDataTypeStr=Inherit: Same as first input
  Switch : Switch  Threshold=1
  Switch1 : Switch  Threshold=1
  Output : Outport
  wires:
  Multiply/1 -> Product2/2
  Switch1/1 -> Output/1
  Constant1/1 -> Switch1/1
  Product2/1 -> Switch1/3
  Switch/1 -> Product2/1
  Divide/1 -> Compare To Zero/1, Switch/3
  Constant2/1 -> Switch/1
  Compare To Zero/1 -> Switch1/2, Switch/2

== system Engine_TestBench/ICE Simple2/Soft ECM/Fuel Consumption/Divide by Zero Fix1 ==
  Divide : Inport
  Multiply : Inport  Port=2
  Compare To Zero : simulink/Logic and Bit Operations/Compare To Zero  relop===  OutDataTypeStr=boolean
  Constant1 : Constant  Value=0
  Constant2 : Constant
  Product2 : Product  Inputs=/*  SaturateOnIntegerOverflow=on  InputSameDT=on  OutDataTypeStr=Inherit: Same as first input
  Switch : Switch  Threshold=1
  Switch1 : Switch  Threshold=1
  Output : Outport
  wires:
  Compare To Zero/1 -> Switch/2, Switch1/2
  Constant2/1 -> Switch/1
  Divide/1 -> Compare To Zero/1, Switch/3
  Switch/1 -> Product2/1
  Product2/1 -> Switch1/3
  Constant1/1 -> Switch1/1
  Switch1/1 -> Output/1
  Multiply/1 -> Product2/2

== system Engine_TestBench/ICE Simple1/Engine Plant Modified/Core Engine/Core Engine/Upstream States ==
  K Converter : nesl_utility/PS-Simulink Converter  PhysicalDomain=network_engine_domain  SubClassName=ps_output  LeftPortType=input  RightPortType=output  PseudoPeriodic=off  Frequencies=[]  Unit=K  AffineConversion=off
  Pa Converter : nesl_utility/PS-Simulink Converter  PhysicalDomain=network_engine_domain  SubClassName=ps_output  LeftPortType=input  RightPortType=output  PseudoPeriodic=off  Frequencies=[]  Unit=Pa  AffineConversion=off
  Pneumatic Absolute Reference : Pneumatic_lib/Pneumatic Elements/Pneumatic Absolute Reference
  Pneumatic Pressure & Temperature Sensor : Pneumatic_lib/Pneumatic Sensors/Pneumatic Pressure & Temperature Sensor
  A : PMIOPort  Port=1  Side=Left
  P (Pa) : Outport
  T (K) : Outport  Port=2
  wires:
  Pa Converter/1 -> P (Pa)/1
  K Converter/1 -> T (K)/1
  connections:
  Pneumatic Pressure & Temperature Sensor/RConn1 -- Pneumatic Absolute Reference/LConn1
  Pneumatic Pressure & Temperature Sensor/LConn1 -- A/RConn1
  K Converter/LConn1 -- Pneumatic Pressure & Temperature Sensor/RConn3
  Pneumatic Pressure & Temperature Sensor/RConn2 -- Pa Converter/LConn1

== system Engine_TestBench/ICE Simple1/Engine Plant Modified/Core Engine/EngEfficiency/Divide by Zero Fix ==
  Multiply : Inport
  Divide : Inport  Port=2
  Compare To Zero : simulink/Logic and Bit Operations/Compare To Zero  relop===  OutDataTypeStr=boolean
  Constant1 : Constant  Value=0
  Constant2 : Constant
  Product2 : Product  Inputs=/*  SaturateOnIntegerOverflow=on  InputSameDT=on  OutDataTypeStr=Inherit: Same as first input
  Switch : Switch  Threshold=1
  Switch1 : Switch  Threshold=1
  Output : Outport
  wires:
  Multiply/1 -> Product2/2
  Switch1/1 -> Output/1
  Constant1/1 -> Switch1/1
  Product2/1 -> Switch1/3
  Switch/1 -> Product2/1
  Divide/1 -> Switch/3, Compare To Zero/1
  Constant2/1 -> Switch/1
  Compare To Zero/1 -> Switch1/2, Switch/2

== system Engine_TestBench/ICE Simple1/Engine Plant Modified/Core Engine/Intake Manifold/Node Potential Sensor ==
  K Converter : nesl_utility/PS-Simulink Converter  PhysicalDomain=network_engine_domain  SubClassName=ps_output  LeftPortType=input  RightPortType=output  PseudoPeriodic=off  Frequencies=[]  Unit=K  AffineConversion=off
  K to C : Fcn  Expr=u(1)-273.15
  Pa Converter : nesl_utility/PS-Simulink Converter  PhysicalDomain=network_engine_domain  SubClassName=ps_output  LeftPortType=input  RightPortType=output  PseudoPeriodic=off  Frequencies=[]  Unit=Pa  AffineConversion=off
  Pa to KPa : Gain  Gain=0.001
  Pneumatic Absolute Reference : Pneumatic_lib/Pneumatic Elements/Pneumatic Absolute Reference
  Pneumatic Pressure & Temperature Sensor : Pneumatic_lib/Pneumatic Sensors/Pneumatic Pressure & Temperature Sensor
  A : PMIOPort  Port=1  Side=Left
  P (KPa) : Outport
  T (C) : Outport  Port=2
  wires:
  Pa Converter/1 -> Pa to KPa/1
  K Converter/1 -> K to C/1
  K to C/1 -> T (C)/1
  Pa to KPa/1 -> P (KPa)/1
  connections:
  Pneumatic Pressure & Temperature Sensor/RConn1 -- Pneumatic Absolute Reference/LConn1
  Pneumatic Pressure & Temperature Sensor/LConn1 -- A/RConn1
  K Converter/LConn1 -- Pneumatic Pressure & Temperature Sensor/RConn3
  Pneumatic Pressure & Temperature Sensor/RConn2 -- Pa Converter/LConn1

== system Engine_TestBench/ICE Simple2/Engine Plant Modified/Core Engine/Core Engine/Upstream States ==
  K Converter : nesl_utility/PS-Simulink Converter  PhysicalDomain=network_engine_domain  SubClassName=ps_output  LeftPortType=input  RightPortType=output  PseudoPeriodic=off  Frequencies=[]  Unit=K  AffineConversion=off
  Pa Converter : nesl_utility/PS-Simulink Converter  PhysicalDomain=network_engine_domain  SubClassName=ps_output  LeftPortType=input  RightPortType=output  PseudoPeriodic=off  Frequencies=[]  Unit=Pa  AffineConversion=off
  Pneumatic Absolute Reference : Pneumatic_lib/Pneumatic Elements/Pneumatic Absolute Reference
  Pneumatic Pressure & Temperature Sensor : Pneumatic_lib/Pneumatic Sensors/Pneumatic Pressure & Temperature Sensor
  A : PMIOPort  Port=1  Side=Left
  P (Pa) : Outport
  T (K) : Outport  Port=2
  wires:
  Pa Converter/1 -> P (Pa)/1
  K Converter/1 -> T (K)/1
  connections:
  Pneumatic Pressure & Temperature Sensor/RConn1 -- Pneumatic Absolute Reference/LConn1
  Pneumatic Pressure & Temperature Sensor/LConn1 -- A/RConn1
  K Converter/LConn1 -- Pneumatic Pressure & Temperature Sensor/RConn3
  Pneumatic Pressure & Temperature Sensor/RConn2 -- Pa Converter/LConn1

== system Engine_TestBench/ICE Simple2/Engine Plant Modified/Core Engine/EngEfficiency/Divide by Zero Fix ==
  Multiply : Inport
  Divide : Inport  Port=2
  Compare To Zero : simulink/Logic and Bit Operations/Compare To Zero  relop===  OutDataTypeStr=boolean
  Constant1 : Constant  Value=0
  Constant2 : Constant
  Product2 : Product  Inputs=/*  SaturateOnIntegerOverflow=on  InputSameDT=on  OutDataTypeStr=Inherit: Same as first input
  Switch : Switch  Threshold=1
  Switch1 : Switch  Threshold=1
  Output : Outport
  wires:
  Multiply/1 -> Product2/2
  Switch1/1 -> Output/1
  Constant1/1 -> Switch1/1
  Product2/1 -> Switch1/3
  Switch/1 -> Product2/1
  Divide/1 -> Switch/3, Compare To Zero/1
  Constant2/1 -> Switch/1
  Compare To Zero/1 -> Switch1/2, Switch/2

== system Engine_TestBench/ICE Simple2/Engine Plant Modified/Core Engine/Intake Manifold/Node Potential Sensor ==
  K Converter : nesl_utility/PS-Simulink Converter  PhysicalDomain=network_engine_domain  SubClassName=ps_output  LeftPortType=input  RightPortType=output  PseudoPeriodic=off  Frequencies=[]  Unit=K  AffineConversion=off
  K to C : Fcn  Expr=u(1)-273.15
  Pa Converter : nesl_utility/PS-Simulink Converter  PhysicalDomain=network_engine_domain  SubClassName=ps_output  LeftPortType=input  RightPortType=output  PseudoPeriodic=off  Frequencies=[]  Unit=Pa  AffineConversion=off
  Pa to KPa : Gain  Gain=0.001
  Pneumatic Absolute Reference : Pneumatic_lib/Pneumatic Elements/Pneumatic Absolute Reference
  Pneumatic Pressure & Temperature Sensor : Pneumatic_lib/Pneumatic Sensors/Pneumatic Pressure & Temperature Sensor
  A : PMIOPort  Port=1  Side=Left
  P (KPa) : Outport
  T (C) : Outport  Port=2
  wires:
  Pa Converter/1 -> Pa to KPa/1
  K Converter/1 -> K to C/1
  K to C/1 -> T (C)/1
  Pa to KPa/1 -> P (KPa)/1
  connections:
  Pneumatic Pressure & Temperature Sensor/RConn1 -- Pneumatic Absolute Reference/LConn1
  Pneumatic Pressure & Temperature Sensor/LConn1 -- A/RConn1
  K Converter/LConn1 -- Pneumatic Pressure & Temperature Sensor/RConn3
  Pneumatic Pressure & Temperature Sensor/RConn2 -- Pa Converter/LConn1

== stateflow chart Engine_TestBench/ICE Simple2/Engine Plant Modified/Core Engine/Crank Process ==
  state Starter_Crank
    du:
    EngActTrq = function(EngSpd_RPM);
  state Eng_Off
    du:
    EngActTrq = 0;
  state Eng_Combustion
    du:
    EngActTrq = 100;
  state CrankTrq = function(EngSpd) [function]
  state Eng_Run
    du:
    EngActTrq = EngBrkTrq;
  (default) -> Eng_Off
  Eng_Off -> Starter_Crank : [EngCrankCmd]
  Starter_Crank -> Eng_Off [order 2] : [!EngCrankCmd]
  Eng_Run -> Eng_Off : [AvlblFuel <= 0.01|| EngShutdown == 1]
  Starter_Crank -> Eng_Combustion [order 1] : after(0.5,sec)
      | [AvlblFuel >= 0.1]
  Eng_Combustion -> Eng_Run : [EngRunAtv]
  data: CrankTrq function_output; EngSpd function_input; EngRunAtv input boolean; AvlblFuel input double; EngActTrq output double; EngCrankCmd input boolean; EngBrkTrq input double; EngSpd_RPM input double; EngShutdown input boolean

== stateflow chart Engine_TestBench/ICE Simple2/Soft ECM/ECM_RollingAliveCnt/Rolling Alive Counter ==
  state RollingAliveCounter
    state Count1
      en: RollingAliveCnt = 0;
    state Count2
      en: RollingAliveCnt = 1;
    state Count3
      en: RollingAliveCnt = 2;
    state Count4
      en: RollingAliveCnt = 3;
    (default) -> Count1
    Count4 -> Count1 : after(0.01,sec)
    Count1 -> Count2 : after(0.01,sec)
    Count2 -> Count3 : after(0.01,sec)
    Count3 -> Count4 : after(0.01,sec)
  data: RollingAliveCnt output int8 =0

== stateflow chart Engine_TestBench/ICE Simple2/Soft ECM/Logic ==
  state Eng_Crank
    en:
    EngCrankCmd = 1;
    FuelPumpEnable = 1;
    EngShutdown = 0;
  state Eng_Off
    en:
    EngRunAtv = 0;
    EngCrankCmd = 0;
    ThrottleCmd = 0;
    FuelPumpEnable = 0;
  state Eng_On
    en:
    EngRunAtv = 1;
    EngCrankCmd = 0;
    du:
    ThrottleCmd = APP2TP(EngSpd_RPM,drvAPP,ShftLvrPos);
  state TP = APP2TP(EngSpd,APP,Shifter) [function]
  (default) -> Eng_Off
  Eng_Off -> Eng_Crank : [SysPwrMd == 3]
  Eng_Crank -> Eng_Off [order 2] : [SysPwrMd < 3]
  Eng_On -> Eng_Off : [SysPwrMd < 2 || EngSpd_RPM < 500]
      | {EngShutdown = 1; }
  Eng_Crank -> Eng_On [order 1] : [EngSpd_RPM >= 580]
  data: EngSpd function_input; TP function_output; APP function_input; Shifter function_input; drvAPP input; ThrottleCmd output double; EngCrankCmd output boolean; SysPwrMd input int8; ShftLvrPos input int8; EngSpd_RPM input double; VehSpdAvgDrvn input double; EngRunAtv output boolean; FuelPumpEnable output double; EngShutdown output boolean

== stateflow chart Engine_TestBench/ICE Simple1/Engine Plant Modified/Core Engine/Crank Process ==
  state Starter_Crank
    du:
    EngActTrq = function(EngSpd_RPM);
  state Eng_Off
    du:
    EngActTrq = 0;
  state Eng_Combustion
    du:
    EngActTrq = 100;
  state CrankTrq = function(EngSpd) [function]
  state Eng_Run
    du:
    EngActTrq = EngBrkTrq;
  (default) -> Eng_Off
  Eng_Off -> Starter_Crank : [EngCrankCmd]
  Starter_Crank -> Eng_Off [order 2] : [!EngCrankCmd]
  Eng_Run -> Eng_Off : [AvlblFuel <= 0.01|| EngShutdown == 1]
  Starter_Crank -> Eng_Combustion [order 1] : after(0.5,sec)
      | [AvlblFuel >= 0.1]
  Eng_Combustion -> Eng_Run : [EngRunAtv]
  data: CrankTrq function_output; EngSpd function_input; EngRunAtv input boolean; AvlblFuel input double; EngActTrq output double; EngCrankCmd input boolean; EngBrkTrq input double; EngSpd_RPM input double; EngShutdown input boolean

== stateflow chart Engine_TestBench/ICE Simple1/Soft ECM/ECM_RollingAliveCnt/Rolling Alive Counter ==
  state RollingAliveCounter
    state Count1
      en: RollingAliveCnt = 0;
    state Count2
      en: RollingAliveCnt = 1;
    state Count3
      en: RollingAliveCnt = 2;
    state Count4
      en: RollingAliveCnt = 3;
    (default) -> Count1
    Count4 -> Count1 : after(0.01,sec)
    Count1 -> Count2 : after(0.01,sec)
    Count2 -> Count3 : after(0.01,sec)
    Count3 -> Count4 : after(0.01,sec)
  data: RollingAliveCnt output int8 =0

== stateflow chart Engine_TestBench/ICE Simple1/Soft ECM/Logic ==
  state Eng_Crank
    en:
    EngCrankCmd = 1;
    FuelPumpEnable = 1;
    EngShutdown = 0;
  state Eng_Off
    en:
    EngRunAtv = 0;
    EngCrankCmd = 0;
    ThrottleCmd = 0;
    FuelPumpEnable = 0;
  state Eng_On
    en:
    EngRunAtv = 1;
    EngCrankCmd = 0;
    du:
    ThrottleCmd = APP2TP(EngSpd_RPM,drvAPP,ShftLvrPos);
  state TP = APP2TP(EngSpd,APP,Shifter) [function]
  (default) -> Eng_Off
  Eng_Off -> Eng_Crank : [SysPwrMd == 3]
  Eng_Crank -> Eng_Off [order 2] : [SysPwrMd < 3]
  Eng_On -> Eng_Off : [SysPwrMd < 2 || EngSpd_RPM < 500]
      | {EngShutdown = 1; }
  Eng_Crank -> Eng_On [order 1] : [EngSpd_RPM >= 580]
  data: EngSpd function_input; TP function_output; APP function_input; Shifter function_input; drvAPP input; ThrottleCmd output double; EngCrankCmd output boolean; SysPwrMd input int8; ShftLvrPos input int8; EngSpd_RPM input double; VehSpdAvgDrvn input double; EngRunAtv output boolean; FuelPumpEnable output double; EngShutdown output boolean
